simulink subsystem "Odometria"  (R2023b)
settings: Solver=VariableStepAuto  StartTime=0.0  StopTime=10.0  RelTol=1e-3
undefined symbols (not defined in the file or in its folder): DiscIntNeverNeededParam
settings Model: Creator=Usuario_UMA  LastModifiedBy=Felix

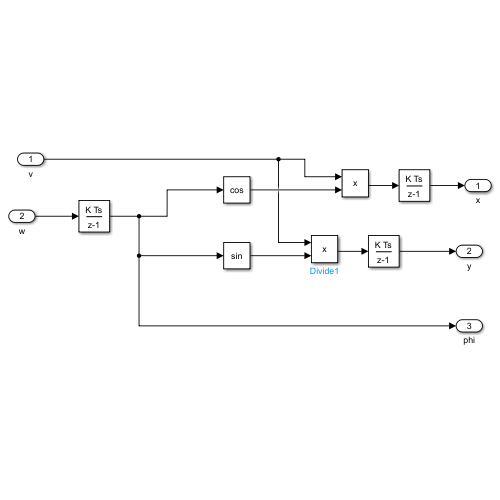
[thumbnail: Simulink's stored preview of the top-level diagram]
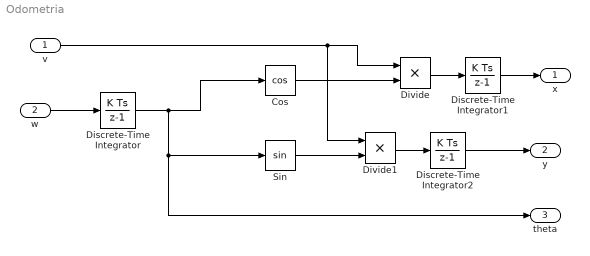
== system Odometria ==
  v : Inport
  w : Inport  Port=2
  Cos : Trigonometry  Operator=cos
  Discrete-Time Integrator : DiscreteIntegrator  SampleTime=0.025  ICPrevOutput=DiscIntNeverNeededParam  ICPrevScaledInput=DiscIntNeverNeededParam
  Discrete-Time Integrator1 : DiscreteIntegrator  SampleTime=0.025  ICPrevOutput=DiscIntNeverNeededParam  ICPrevScaledInput=DiscIntNeverNeededParam
  Discrete-Time Integrator2 : DiscreteIntegrator  SampleTime=0.025  ICPrevOutput=DiscIntNeverNeededParam  ICPrevScaledInput=DiscIntNeverNeededParam
  Divide : Product  Inputs=**
  Divide1 : Product  Inputs=**
  Sin : Trigonometry
  x : Outport
  y : Outport  Port=2
  theta : Outport  Port=3
  wires:
  w/1 -> Discrete-Time Integrator/1
  Cos/1 -> Divide/2
  v/1 -> Divide1/1, Divide/1
  Divide/1 -> Discrete-Time Integrator1/1
  Discrete-Time Integrator1/1 -> x/1
  Divide1/1 -> Discrete-Time Integrator2/1
  Sin/1 -> Divide1/2
  Discrete-Time Integrator2/1 -> y/1
  Discrete-Time Integrator/1 -> Sin/1, theta/1, Cos/1
